simulink library "DEMDlib"  (R2024a)
settings: Solver=VariableStepAuto  StartTime=0.0  StopTime=10.0  RelTol=1e-3
values from neighbouring files (symbols this model uses):
  Lks = Ls - Lm*k    (= 0.00442538071066)    [parameters.m]
  np = 3    [parameters.m]
  Rs = 0.24    [parameters.m]
libraries: $bdroot x3, eeGeneralControl x1
settings Model: Creator=roberto  LastModifiedBy=roberto

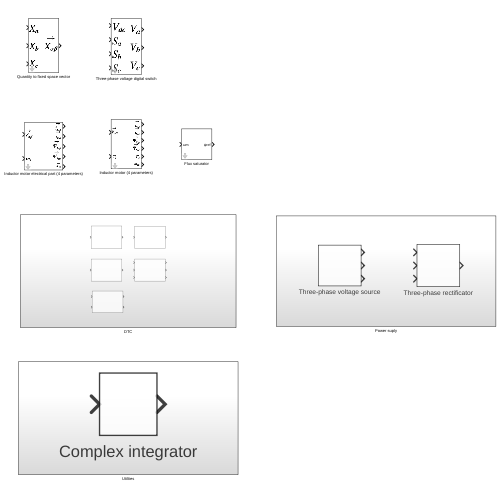
[thumbnail: Simulink's stored preview of the top-level diagram]
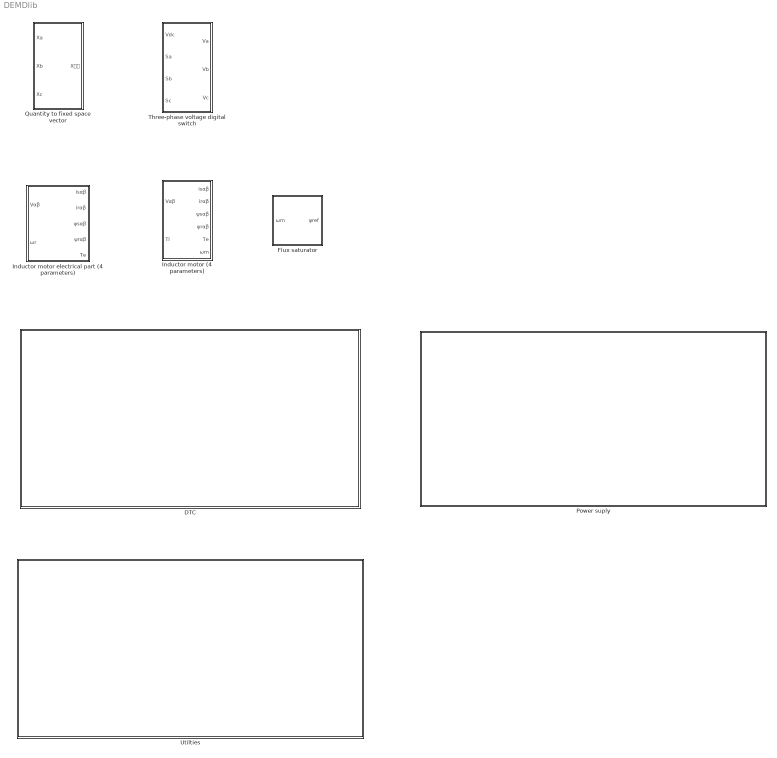
== system DEMDlib ==
  DTC : Subsystem
  Flux saturator : Subsystem  mask(Flux saturator){psin=0, wmb=0}
      mask DialogControl Control3 Prompt: Base speed (rad/s)
      mask DialogControl Control2 Prompt: Nominal flux
      mask DialogControl Control4 Prompt: Base speed
  Inductor motor (4 parameters) : Subsystem  mask(Inductor motor (4 parameters)){Rs=0, Lks=0, Rr=0, Lm=0, np=3, J=0, B=0}
      mask DialogControl ParameterGroupVar Prompt: Eletrical parameters
      mask DialogControl Control2 Prompt: Stator resistance (Rs)
      mask DialogControl Control3 Prompt: Stator equivalent inductance (Lks)
      mask DialogControl Control4 Prompt: Rotor resistance (Rr)
      mask DialogControl Control5 Prompt: Mutual inducatance (Lm)
      mask DialogControl Control6 Prompt: Number of poles (np)
      mask DialogControl ParameterGroupVar_copy Prompt: Mechanical parameters
      mask DialogControl Control7 Prompt: Motor moment of inertia (J)
      mask DialogControl Control8 Prompt: Viscous friction coefficient (B)
  Inductor motor electrical part (4 parameters) : Subsystem  mask(Inductor motor electrical part (4 parameters)){Rs=0, Lks=0, Rr=0, Lm=0, np=3}
      mask DialogControl ParameterGroupVar Prompt: Eletrical parameters
      mask DialogControl Control2 Prompt: Stator resistance (Rs)
      mask DialogControl Control3 Prompt: Stator equivalent inductance (Lks)
      mask DialogControl Control4 Prompt: Rotor resistance (Rr)
      mask DialogControl Control5 Prompt: Mutual inducatance (Lm)
      mask DialogControl Control6 Prompt: Number of poles (np)
  Power suply : Subsystem
  Quantity to fixed space vector : Subsystem  mask(Quantity to fixed space vector){}
  Three-phase voltage digital switch : Subsystem  mask(Three-phase voltage digital switch){}
  Utilties : Subsystem

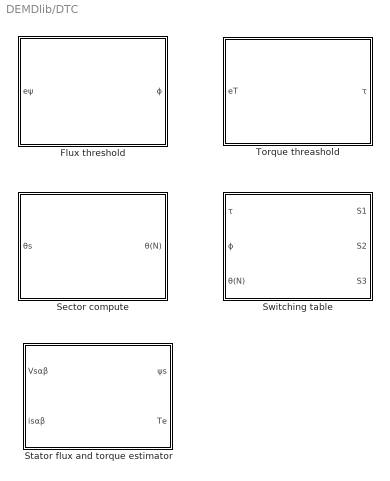
== system DEMDlib/DTC ==
  Flux threshold : Subsystem  mask(Flux threashold){dpsi=1}
      mask DialogControl Control2 Prompt: Δψ
  Sector compute : Subsystem  mask(Sector compute){}
  Stator flux and torque estimator : Subsystem  mask(Stator flux and torque estimator){Rs=Rs, Lks=Lks, np=np, a=2}
      mask DialogControl Control2 Prompt: Stator resistance (Rs)
      mask DialogControl Control3 Prompt: Stator equivalent inductance (Lks)
      mask DialogControl Control4 Prompt: Number of poles (np)
      mask DialogControl Container3 Prompt: Filter parameters
      mask DialogControl Control5 Prompt: Filter time costant
  Switching table : Subsystem  mask(Switching table){}
  Torque threashold : Subsystem  mask(Torque threashold){dT=1}
      mask DialogControl Control2 Prompt: ΔT

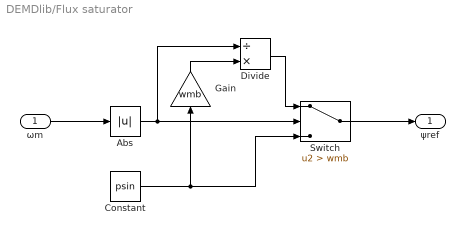
== system DEMDlib/Flux saturator ==
  ωm : Inport
  Abs : Abs  SaturateOnIntegerOverflow=off
  Constant : Constant  Value=psin
  Divide : Product  Inputs=/*
  Gain : Gain  Gain=wmb
  Switch : Switch  Criteria=u2 > Threshold  Threshold=wmb  SaturateOnIntegerOverflow=off  InputSameDT=off
  ψref : Outport
  wires:
  Constant/1 -> Switch/3, Gain/1
  ωm/1 -> Abs/1
  Switch/1 -> ψref/1
  Abs/1 -> Divide/1, Switch/2
  Divide/1 -> Switch/1
  Gain/1 -> Divide/2

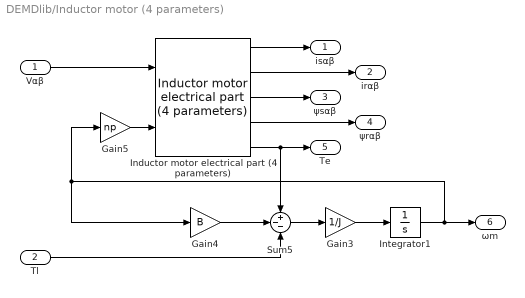
== system DEMDlib/Inductor motor (4 parameters) ==
  Vαβ : Inport
  Tl : Inport  Port=2
  Gain3 : Gain  Gain=1/J
  Gain4 : Gain  Gain=B
  Gain5 : Gain  Gain=np
  Inductor motor electrical part (4 parameters) : $bdroot/Inductor motor electrical part (4 parameters)  Rs=Rs  Lks=Lks  Rr=Rr  Lm=Lm  np=np
  Integrator1 : Integrator
  Sum5 : Sum  Inputs=+--
  isαβ : Outport
  irαβ : Outport  Port=2
  ψsαβ : Outport  Port=3
  ψrαβ : Outport  Port=4
  Te : Outport  Port=5
  ωm : Outport  Port=6
  wires:
  Tl/1 -> Sum5/3
  Inductor motor electrical part (4 parameters)/5 -> Te/1, Sum5/1
  Integrator1/1 -> Gain4/1, Gain5/1, ωm/1
  Sum5/1 -> Gain3/1
  Gain3/1 -> Integrator1/1
  Gain4/1 -> Sum5/2
  Vαβ/1 -> Inductor motor electrical part (4 parameters)/1
  Inductor motor electrical part (4 parameters)/3 -> ψsαβ/1
  Inductor motor electrical part (4 parameters)/1 -> isαβ/1
  Inductor motor electrical part (4 parameters)/2 -> irαβ/1
  Inductor motor electrical part (4 parameters)/4 -> ψrαβ/1
  Gain5/1 -> Inductor motor electrical part (4 parameters)/2

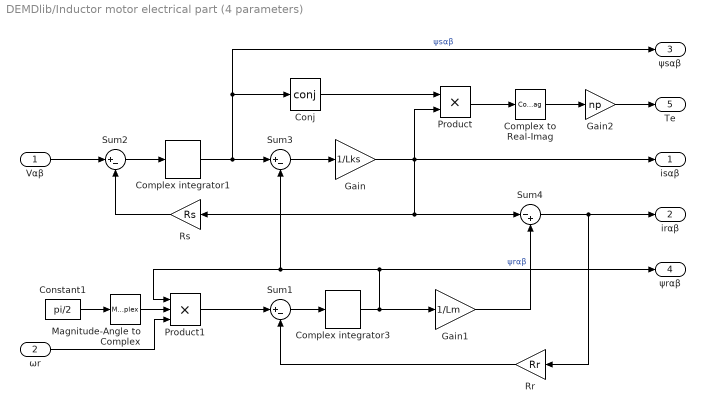
== system DEMDlib/Inductor motor electrical part (4 parameters) ==
  Vαβ : Inport
  ωr : Inport  Port=2
  Complex integrator1 : $bdroot/Utilties/Complex integrator
  Complex integrator3 : $bdroot/Utilties/Complex integrator
  Complex to Real-Imag : ComplexToRealImag  Output=Imag
  Conj : Math  Operator=conj
  Constant1 : Constant  Value=pi/2
  Gain : Gain  Gain=1/Lks
  Gain1 : Gain  Gain=1/Lm
  Gain2 : Gain  Gain=np
  Magnitude-Angle to Complex : MagnitudeAngleToComplex  Input=Angle  ConstantPart=1
  Product : Product
  Product1 : Product  Inputs=3
  Rr : Gain  Gain=Rr
  Rs : Gain  Gain=Rs
  Sum1 : Sum  Inputs=|+-
  Sum2 : Sum  Inputs=|+-
  Sum3 : Sum  Inputs=|+-
  Sum4 : Sum  Inputs=|-+
  isαβ : Outport
  irαβ : Outport  Port=2
  ψsαβ : Outport  Port=3
  ψrαβ : Outport  Port=4
  Te : Outport  Port=5
  wires:
  Gain1/1 -> Sum4/2
  Rs/1 -> Sum2/2
  Complex to Real-Imag/1 -> Gain2/1
  Product/1 -> Complex to Real-Imag/1
  Complex integrator1/1 -> ψsαβ/1, Conj/1, Sum3/1  "ψsαβ"
  Gain/1 -> isαβ/1, Product/2, Sum4/1, Rs/1
  Sum4/1 -> Rr/1, irαβ/1
  Vαβ/1 -> Sum2/1
  Gain2/1 -> Te/1
  Sum2/1 -> Complex integrator1/1
  Conj/1 -> Product/1
  Sum3/1 -> Gain/1
  Complex integrator3/1 -> Gain1/1, Sum3/2, Product1/1, ψrαβ/1  "ψrαβ"
  Sum1/1 -> Complex integrator3/1
  Rr/1 -> Sum1/2
  ωr/1 -> Product1/3
  Constant1/1 -> Magnitude-Angle to Complex/1
  Magnitude-Angle to Complex/1 -> Product1/2
  Product1/1 -> Sum1/1

== system DEMDlib/Power suply ==
  Three-phase rectificator : Subsystem  mask(Three-phase rectifier){}
  Three-phase voltage source : Subsystem  mask(Three-phase voltage source){Vac=230, fac=50*2*pi}
      mask DialogControl Control2 Prompt: Line voltage
      mask DialogControl Control3 Prompt: Voltage frequency (rad/s)

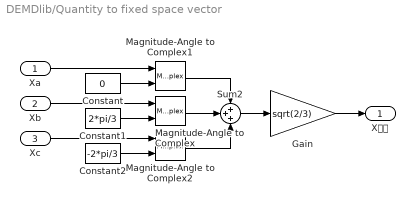
== system DEMDlib/Quantity to fixed space vector ==
  Xa : Inport
  Xb : Inport  Port=2
  Xc : Inport  Port=3
  Constant : Constant  Value=0
  Constant1 : Constant  Value=2*pi/3
  Constant2 : Constant  Value=-2*pi/3
  Gain : Gain  Gain=sqrt(2/3)
  Magnitude-Angle to Complex : MagnitudeAngleToComplex
  Magnitude-Angle to Complex1 : MagnitudeAngleToComplex
  Magnitude-Angle to Complex2 : MagnitudeAngleToComplex
  Sum2 : Sum  Inputs=+++
  X𝛼𝛽 : Outport
  wires:
  Constant1/1 -> Magnitude-Angle to Complex/2
  Constant2/1 -> Magnitude-Angle to Complex2/2
  Xc/1 -> Magnitude-Angle to Complex2/1
  Constant/1 -> Magnitude-Angle to Complex1/2
  Magnitude-Angle to Complex1/1 -> Sum2/1
  Magnitude-Angle to Complex/1 -> Sum2/2
  Xb/1 -> Magnitude-Angle to Complex/1
  Magnitude-Angle to Complex2/1 -> Sum2/3
  Sum2/1 -> Gain/1
  Xa/1 -> Magnitude-Angle to Complex1/1
  Gain/1 -> X𝛼𝛽/1

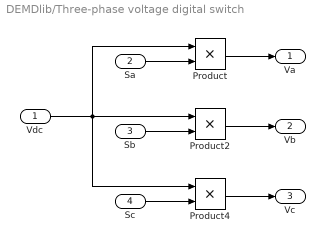
== system DEMDlib/Three-phase voltage digital switch ==
  Vdc : Inport
  Sa : Inport  Port=2
  Sb : Inport  Port=3
  Sc : Inport  Port=4
  Product : Product
  Product2 : Product
  Product4 : Product
  Va : Outport
  Vb : Outport  Port=2
  Vc : Outport  Port=3
  wires:
  Product4/1 -> Vc/1
  Product/1 -> Va/1
  Product2/1 -> Vb/1
  Sa/1 -> Product/2
  Sb/1 -> Product2/2
  Sc/1 -> Product4/2
  Vdc/1 -> Product4/1, Product/1, Product2/1

== system DEMDlib/Utilties ==
  Complex integrator : Subsystem
      mask Display: droots([],0,1);

== system DEMDlib/DTC/Flux threshold ==
  eψ : Inport
  Relay : Relay  OnSwitchValue=dpsi  OffSwitchValue=-dpsi
  ϕ : Outport
  wires:
  Relay/1 -> ϕ/1
  eψ/1 -> Relay/1

== system DEMDlib/DTC/Sector compute ==
  θs : Inport
  MATLAB Function : MATLAB Function  TreatAsAtomicUnit=on
  θ(N) : Outport
  wires:
  θs/1 -> MATLAB Function/1(theta)
  MATLAB Function/1(thetaN) -> θ(N)/1

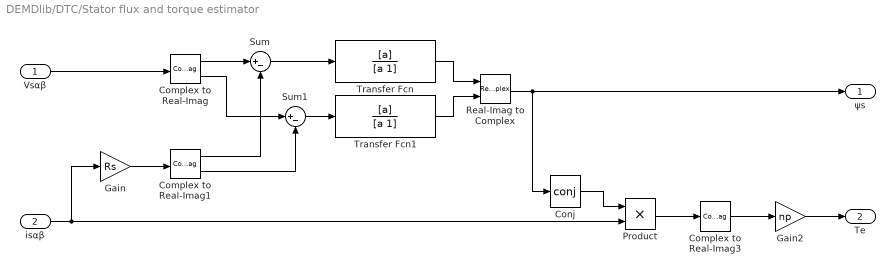
== system DEMDlib/DTC/Stator flux and torque estimator ==
  Vsαβ : Inport
  isαβ : Inport  Port=2
  Complex to Real-Imag : ComplexToRealImag
  Complex to Real-Imag1 : ComplexToRealImag
  Complex to Real-Imag3 : ComplexToRealImag  Output=Imag
  Conj : Math  Operator=conj
  Gain : Gain  Gain=Rs
  Gain2 : Gain  Gain=np
  Product : Product
  Real-Imag to Complex : RealImagToComplex
  Sum : Sum  Inputs=|+-
  Sum1 : Sum  Inputs=|+-
  Transfer Fcn : TransferFcn  Numerator=[a]  Denominator=[a 1]
  Transfer Fcn1 : TransferFcn  Numerator=[a]  Denominator=[a 1]
  ψs : Outport
  Te : Outport  Port=2
  wires:
  Vsαβ/1 -> Complex to Real-Imag/1
  isαβ/1 -> Product/2, Gain/1
  Gain/1 -> Complex to Real-Imag1/1
  Complex to Real-Imag/1 -> Sum/1
  Complex to Real-Imag/2 -> Sum1/1
  Complex to Real-Imag1/1 -> Sum/2
  Complex to Real-Imag1/2 -> Sum1/2
  Transfer Fcn1/1 -> Real-Imag to Complex/2
  Transfer Fcn/1 -> Real-Imag to Complex/1
  Real-Imag to Complex/1 -> ψs/1, Conj/1
  Gain2/1 -> Te/1
  Conj/1 -> Product/1
  Product/1 -> Complex to Real-Imag3/1
  Complex to Real-Imag3/1 -> Gain2/1
  Sum/1 -> Transfer Fcn/1
  Sum1/1 -> Transfer Fcn1/1

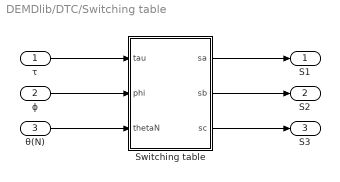
== system DEMDlib/DTC/Switching table ==
  τ : Inport
  ϕ : Inport  Port=2
  θ(N) : Inport  Port=3
  Switching table : MATLAB Function  TreatAsAtomicUnit=on
  S1 : Outport
  S2 : Outport  Port=2
  S3 : Outport  Port=3
  wires:
  θ(N)/1 -> Switching table/3(thetaN)
  Switching table/1(sa) -> S1/1
  Switching table/3(sc) -> S3/1
  Switching table/2(sb) -> S2/1
  ϕ/1 -> Switching table/2(phi)
  τ/1 -> Switching table/1(tau)

== system DEMDlib/DTC/Torque threashold ==
  eT : Inport
  CCW : Relay  OnSwitchValue=dT  OffSwitchValue=0
  CW : Relay  OnSwitchValue=0  OffSwitchValue=-dT  OnOutputValue=0  OffOutputValue=-1
  Sum : Sum  Inputs=|++
  τ : Outport
  wires:
  Sum/1 -> τ/1
  eT/1 -> CW/1, CCW/1
  CW/1 -> Sum/2
  CCW/1 -> Sum/1

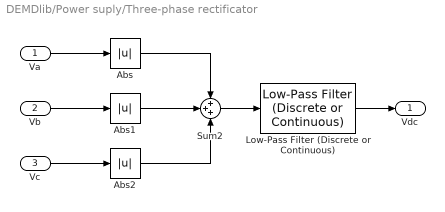
== system DEMDlib/Power suply/Three-phase rectificator ==
  Va : Inport
  Vb : Inport  Port=2
  Vc : Inport  Port=3
  Abs : Abs  SaturateOnIntegerOverflow=off
  Abs1 : Abs  SaturateOnIntegerOverflow=off
  Abs2 : Abs  SaturateOnIntegerOverflow=off
  Low-Pass Filter (Discrete or Continuous) : eeGeneralControl/Low-Pass Filter (Discrete or Continuous)  K=1  T=1/(50*2*pi)  B=inf  A=-inf  init_option=Inherited from block input  x0=0  Ts=0
  Sum2 : Sum  Inputs=+++
  Vdc : Outport
  wires:
  Abs2/1 -> Sum2/3
  Low-Pass Filter (Discrete or Continuous)/1 -> Vdc/1
  Abs1/1 -> Sum2/2
  Sum2/1 -> Low-Pass Filter (Discrete or Continuous)/1
  Vc/1 -> Abs2/1
  Vb/1 -> Abs1/1
  Va/1 -> Abs/1
  Abs/1 -> Sum2/1

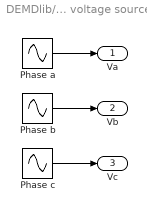
== system DEMDlib/Power suply/Three-phase voltage source ==
  Phase a : Sin  Amplitude=Vac  Frequency=fac  SampleTime=0
  Phase b : Sin  Amplitude=Vac  Frequency=fac  Phase=-2*pi/3  SampleTime=0
  Phase c : Sin  Amplitude=Vac  Frequency=fac  Phase=-4*pi/3  SampleTime=0
  Va : Outport
  Vb : Outport  Port=2
  Vc : Outport  Port=3
  wires:
  Phase a/1 -> Va/1
  Phase c/1 -> Vc/1
  Phase b/1 -> Vb/1

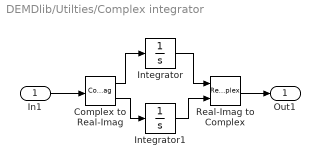
== system DEMDlib/Utilties/Complex integrator ==
  In1 : Inport
  Complex to Real-Imag : ComplexToRealImag
  Integrator : Integrator
  Integrator1 : Integrator
  Real-Imag to Complex : RealImagToComplex
  Out1 : Outport
  wires:
  In1/1 -> Complex to Real-Imag/1
  Real-Imag to Complex/1 -> Out1/1
  Integrator1/1 -> Real-Imag to Complex/2
  Integrator/1 -> Real-Imag to Complex/1
  Complex to Real-Imag/1 -> Integrator/1
  Complex to Real-Imag/2 -> Integrator1/1

== matlab function DEMDlib/DTC/Sector compute/MATLAB Function ==
  data: theta input; thetaN output
function thetaN = fcn(theta)

sector_number = 6;
sector_size = 2*pi / sector_number;
first_sector_offset = sector_size /2;

% move first sector start from -first_sector_offset to 0
theta = theta + first_sector_offset;

theta = rem(theta, 2*pi);

% make theta always positive
theta = theta + (theta < 0) * 2*pi;

thetaN = floor(theta /sector_size) + 1;

% prevent overflow due to numerical errors
thetaN = thetaN - (thetaN > sector_number) * sector_number;

== matlab function DEMDlib/DTC/Switching table/Switching table ==
  data: tau input; phi input; sa output; thetaN input; sb output; sc output
function [sa,sb,sc]= fcn(tau,phi,thetaN)

phi = ((phi > 0.5) * 1) + 1;
tau = ((tau > 0.5) * 1 + (tau < -0.5) * -1) + 2;

% T(phi+1, tau+2, thetaN, V)
T = zeros(2,3,6,3);

T(1,3,1,:) = [0 1 0];
T(1,2,1,:) = [0 0 0];
T(1,1,1,:) = [0 0 1];
T(2,3,1,:) = [1 1 0];
T(2,2,1,:) = [1 1 1];
T(2,1,1,:) = [1 0 1];

T(1,3,2,:) = [0 1 1];
T(1,2,2,:) = [1 1 1];
T(1,1,2,:) = [1 0 1];
T(2,3,2,:) = [0 1 0];
T(2,2,2,:) = [0 0 0];
T(2,1,2,:) = [1 0 0];

T(1,3,3,:) = [0 0 1];
T(1,2,3,:) = [0 0 0];
T(1,1,3,:) = [1 0 0];
T(2,3,3,:) = [0 1 1];
T(2,2,3,:) = [1 1 1];
T(2,1,3,:) = [1 1 0];

T(1,3,4,:) = [1 0 1];
T(1,2,4,:) = [1 1 1];
T(1,1,4,:) = [1 1 0];
T(2,3,4,:) = [0 0 1];
T(2,2,4,:) = [0 0 0];
T(2,1,4,:) = [0 1 0];

T(1,3,5,:) = [1 0 0];
T(1,2,5,:) = [0 0 0];
T(1,1,5,:) = [0 1 0];
T(2,3,5,:) = [1 0 1];
T(2,2,5,:) = [1 1 1];
T(2,1,5,:) = [0 1 1];

T(1,3,6,:) = [1 1 0];
T(1,2,6,:) = [1 1 1];
T(1,1,6,:) = [0 1 1];
T(2,3,6,:) = [1 0 0];
T(2,2,6,:) = [0 0 0];
T(2,1,6,:) = [0 0 1];

S = squeeze(T(phi, tau, thetaN,:));

sa = S(1);
sb = S(2);
sc = S(3);
